simulink model "PI_PSO"  (R2021a)
settings: Solver=VariableStepAuto  StartTime=0.0  StopTime=100  RelTol=1e-6  AbsTol=1e-6
undefined symbols (not defined in the file or in its folder): DiscIntNeverNeededParam, G, Solar_time, wind, wind_time
libraries: powerlib_extras x24, pid_lib x6, simulink x2
(part 2 of 2)

== system PI_PSO/AREA 2/Performance Indices/ITSE ==
  In1 : Inport
  Clock : Clock
  Discrete-Time Integrator : DiscreteIntegrator  gainval=1  SampleTime=-1  ICPrevOutput=DiscIntNeverNeededParam  ICPrevScaledInput=DiscIntNeverNeededParam
  Divide : Product  Inputs=**
  Math Function : Math  Operator=square  SignedPower=on  SaturateOnIntegerOverflow=on
  Out1 : Outport
  wires:
  Discrete-Time Integrator/1 -> Out1/1
  In1/1 -> Math Function/1
  Divide/1 -> Discrete-Time Integrator/1
  Math Function/1 -> Divide/1
  Clock/1 -> Divide/2

== system PI_PSO/AREA 2/Performance Indices/Subsystem1 ==
  In1 : Inport
  Id_ref step : powerlib_extras/Control  Blocks/Timer  t=[0 1]  e=[0 1]
      settings: SourceProductBaseCode=PS
  Prod : Product  InputSameDT=on  SaturateOnIntegerOverflow=on  OutDataTypeStr=Inherit: Same as first input
  DP1 : Outport
  wires:
  Id_ref step/1 -> Prod/2
  In1/1 -> Prod/1
  Prod/1 -> DP1/1

== system PI_PSO/AREA 2/Performance Indices/Subsystem2 ==
  In1 : Inport
  Id_ref step : powerlib_extras/Control  Blocks/Timer  t=[0 1]  e=[0 1]
      settings: SourceProductBaseCode=PS
  Prod : Product  InputSameDT=on  SaturateOnIntegerOverflow=on  OutDataTypeStr=Inherit: Same as first input
  Out1 : Outport
  wires:
  Id_ref step/1 -> Prod/2
  In1/1 -> Prod/1
  Prod/1 -> Out1/1

== system PI_PSO/AREA 2/Performance Indices/Subsystem3 ==
  In1 : Inport
  Id_ref step : powerlib_extras/Control  Blocks/Timer  t=[0 1]  e=[0 1]
      settings: SourceProductBaseCode=PS
  Prod : Product  InputSameDT=on  SaturateOnIntegerOverflow=on  OutDataTypeStr=Inherit: Same as first input
  Out1 : Outport
  wires:
  Prod/1 -> Out1/1
  In1/1 -> Prod/1
  Id_ref step/1 -> Prod/2

== system PI_PSO/AREA 2/Performance Indices/Subsystem5 ==
  In1 : Inport
  Id_ref step : powerlib_extras/Control  Blocks/Timer  t=[0 1]  e=[0 1]
      settings: SourceProductBaseCode=PS
  Prod : Product  InputSameDT=on  SaturateOnIntegerOverflow=on  OutDataTypeStr=Inherit: Same as first input
  Out1 : Outport
  wires:
  Prod/1 -> Out1/1
  In1/1 -> Prod/1
  Id_ref step/1 -> Prod/2

== system PI_PSO/AREA 3/Performance Indices/IAE ==
  In1 : Inport
  Abs : Abs
  Discrete-Time Integrator : DiscreteIntegrator  gainval=1  SampleTime=-1  ICPrevOutput=DiscIntNeverNeededParam  ICPrevScaledInput=DiscIntNeverNeededParam
  Out1 : Outport
  wires:
  Abs/1 -> Discrete-Time Integrator/1
  Discrete-Time Integrator/1 -> Out1/1
  In1/1 -> Abs/1

== system PI_PSO/AREA 3/Performance Indices/ISE ==
  In1 : Inport
  Discrete-Time Integrator : DiscreteIntegrator  gainval=1  SampleTime=-1  ICPrevOutput=DiscIntNeverNeededParam  ICPrevScaledInput=DiscIntNeverNeededParam
  Math Function : Math  Operator=square  SignedPower=on  SaturateOnIntegerOverflow=on
  Out1 : Outport
  wires:
  In1/1 -> Math Function/1
  Discrete-Time Integrator/1 -> Out1/1
  Math Function/1 -> Discrete-Time Integrator/1

== system PI_PSO/AREA 3/Performance Indices/ITAE2 ==
  In1 : Inport
  Abs : Abs
  Clock : Clock
  Discrete-Time Integrator : DiscreteIntegrator  gainval=1  SampleTime=-1  ICPrevOutput=DiscIntNeverNeededParam  ICPrevScaledInput=DiscIntNeverNeededParam
  Divide : Product  Inputs=**
  Out1 : Outport
  wires:
  Clock/1 -> Divide/2
  Abs/1 -> Divide/1
  Divide/1 -> Discrete-Time Integrator/1
  In1/1 -> Abs/1
  Discrete-Time Integrator/1 -> Out1/1

== system PI_PSO/AREA 3/Performance Indices/ITSE ==
  In1 : Inport
  Clock : Clock
  Discrete-Time Integrator : DiscreteIntegrator  gainval=1  SampleTime=-1  ICPrevOutput=DiscIntNeverNeededParam  ICPrevScaledInput=DiscIntNeverNeededParam
  Divide : Product  Inputs=**
  Math Function : Math  Operator=square  SignedPower=on  SaturateOnIntegerOverflow=on
  Out1 : Outport
  wires:
  Discrete-Time Integrator/1 -> Out1/1
  In1/1 -> Math Function/1
  Divide/1 -> Discrete-Time Integrator/1
  Math Function/1 -> Divide/1
  Clock/1 -> Divide/2

== system PI_PSO/AREA 3/Performance Indices/Subsystem1 ==
  In1 : Inport
  Id_ref step : powerlib_extras/Control  Blocks/Timer  t=[0 1]  e=[0 1]
      settings: SourceProductBaseCode=PS
  Prod : Product  InputSameDT=on  SaturateOnIntegerOverflow=on  OutDataTypeStr=Inherit: Same as first input
  Out1 : Outport
  wires:
  Id_ref step/1 -> Prod/2
  In1/1 -> Prod/1
  Prod/1 -> Out1/1

== system PI_PSO/AREA 3/Performance Indices/Subsystem2 ==
  In1 : Inport
  Id_ref step : powerlib_extras/Control  Blocks/Timer  t=[0 1]  e=[0 1]
      settings: SourceProductBaseCode=PS
  Prod : Product  InputSameDT=on  SaturateOnIntegerOverflow=on  OutDataTypeStr=Inherit: Same as first input
  DP1 : Outport
  wires:
  Id_ref step/1 -> Prod/2
  In1/1 -> Prod/1
  Prod/1 -> DP1/1

== system PI_PSO/AREA 3/Performance Indices/Subsystem3 ==
  In1 : Inport
  Id_ref step : powerlib_extras/Control  Blocks/Timer  t=[0 1]  e=[0 1]
      settings: SourceProductBaseCode=PS
  Prod : Product  InputSameDT=on  SaturateOnIntegerOverflow=on  OutDataTypeStr=Inherit: Same as first input
  Out1 : Outport
  wires:
  Prod/1 -> Out1/1
  In1/1 -> Prod/1
  Id_ref step/1 -> Prod/2

== system PI_PSO/AREA 3/Performance Indices/Subsystem5 ==
  In1 : Inport
  Id_ref step : powerlib_extras/Control  Blocks/Timer  t=[0 1]  e=[0 1]
      settings: SourceProductBaseCode=PS
  Prod : Product  InputSameDT=on  SaturateOnIntegerOverflow=on  OutDataTypeStr=Inherit: Same as first input
  Out1 : Outport
  wires:
  Prod/1 -> Out1/1
  In1/1 -> Prod/1
  Id_ref step/1 -> Prod/2

== system PI_PSO/AREA 4/Performance Indices/IAE ==
  In1 : Inport
  Abs : Abs
  Discrete-Time Integrator : DiscreteIntegrator  gainval=1  SampleTime=-1  ICPrevOutput=DiscIntNeverNeededParam  ICPrevScaledInput=DiscIntNeverNeededParam
  Out1 : Outport
  wires:
  Abs/1 -> Discrete-Time Integrator/1
  Discrete-Time Integrator/1 -> Out1/1
  In1/1 -> Abs/1

== system PI_PSO/AREA 4/Performance Indices/ISE ==
  In1 : Inport
  Discrete-Time Integrator : DiscreteIntegrator  gainval=1  SampleTime=-1  ICPrevOutput=DiscIntNeverNeededParam  ICPrevScaledInput=DiscIntNeverNeededParam
  Math Function : Math  Operator=square  SignedPower=on  SaturateOnIntegerOverflow=on
  Out1 : Outport
  wires:
  In1/1 -> Math Function/1
  Discrete-Time Integrator/1 -> Out1/1
  Math Function/1 -> Discrete-Time Integrator/1

== system PI_PSO/AREA 4/Performance Indices/ITAE4 ==
  In1 : Inport
  Abs : Abs
  Clock : Clock
  Discrete-Time Integrator : DiscreteIntegrator  gainval=1  SampleTime=-1  ICPrevOutput=DiscIntNeverNeededParam  ICPrevScaledInput=DiscIntNeverNeededParam
  Divide : Product  Inputs=**
  Out1 : Outport
  wires:
  Clock/1 -> Divide/2
  Abs/1 -> Divide/1
  Divide/1 -> Discrete-Time Integrator/1
  In1/1 -> Abs/1
  Discrete-Time Integrator/1 -> Out1/1

== system PI_PSO/AREA 4/Performance Indices/ITSE ==
  In1 : Inport
  Clock : Clock
  Discrete-Time Integrator : DiscreteIntegrator  gainval=1  SampleTime=-1  ICPrevOutput=DiscIntNeverNeededParam  ICPrevScaledInput=DiscIntNeverNeededParam
  Divide : Product  Inputs=**
  Math Function : Math  Operator=square  SignedPower=on  SaturateOnIntegerOverflow=on
  Out1 : Outport
  wires:
  Discrete-Time Integrator/1 -> Out1/1
  In1/1 -> Math Function/1
  Divide/1 -> Discrete-Time Integrator/1
  Math Function/1 -> Divide/1
  Clock/1 -> Divide/2

== system PI_PSO/AREA 4/Performance Indices/Subsystem1 ==
  In1 : Inport
  Id_ref step : powerlib_extras/Control  Blocks/Timer  t=[0 1]  e=[0 1]
      settings: SourceProductBaseCode=PS
  Prod : Product  InputSameDT=on  SaturateOnIntegerOverflow=on  OutDataTypeStr=Inherit: Same as first input
  Out1 : Outport
  wires:
  Id_ref step/1 -> Prod/2
  In1/1 -> Prod/1
  Prod/1 -> Out1/1

== system PI_PSO/AREA 4/Performance Indices/Subsystem2 ==
  In1 : Inport
  Id_ref step : powerlib_extras/Control  Blocks/Timer  t=[0 1]  e=[0 1]
      settings: SourceProductBaseCode=PS
  Prod : Product  InputSameDT=on  SaturateOnIntegerOverflow=on  OutDataTypeStr=Inherit: Same as first input
  Out1 : Outport
  wires:
  Prod/1 -> Out1/1
  In1/1 -> Prod/1
  Id_ref step/1 -> Prod/2

== system PI_PSO/AREA 4/Performance Indices/Subsystem3 ==
  In1 : Inport
  Id_ref step : powerlib_extras/Control  Blocks/Timer  t=[0 1]  e=[0 1]
      settings: SourceProductBaseCode=PS
  Prod : Product  InputSameDT=on  SaturateOnIntegerOverflow=on  OutDataTypeStr=Inherit: Same as first input
  DP1 : Outport
  wires:
  Id_ref step/1 -> Prod/2
  In1/1 -> Prod/1
  Prod/1 -> DP1/1

== system PI_PSO/AREA 4/Performance Indices/Subsystem5 ==
  In1 : Inport
  Id_ref step : powerlib_extras/Control  Blocks/Timer  t=[0 1]  e=[0 1]
      settings: SourceProductBaseCode=PS
  Prod : Product  InputSameDT=on  SaturateOnIntegerOverflow=on  OutDataTypeStr=Inherit: Same as first input
  Out1 : Outport
  wires:
  Prod/1 -> Out1/1
  In1/1 -> Prod/1
  Id_ref step/1 -> Prod/2

== system PI_PSO/AREA 5/Performance Indices/IAE ==
  In1 : Inport
  Abs : Abs
  Discrete-Time Integrator : DiscreteIntegrator  gainval=1  SampleTime=-1  ICPrevOutput=DiscIntNeverNeededParam  ICPrevScaledInput=DiscIntNeverNeededParam
  Out1 : Outport
  wires:
  Abs/1 -> Discrete-Time Integrator/1
  Discrete-Time Integrator/1 -> Out1/1
  In1/1 -> Abs/1

== system PI_PSO/AREA 5/Performance Indices/ISE ==
  In1 : Inport
  Discrete-Time Integrator : DiscreteIntegrator  gainval=1  SampleTime=-1  ICPrevOutput=DiscIntNeverNeededParam  ICPrevScaledInput=DiscIntNeverNeededParam
  Math Function : Math  Operator=square  SignedPower=on  SaturateOnIntegerOverflow=on
  Out1 : Outport
  wires:
  In1/1 -> Math Function/1
  Discrete-Time Integrator/1 -> Out1/1
  Math Function/1 -> Discrete-Time Integrator/1

== system PI_PSO/AREA 5/Performance Indices/ITAE5 ==
  In1 : Inport
  Abs : Abs
  Clock : Clock
  Discrete-Time Integrator : DiscreteIntegrator  gainval=1  SampleTime=-1  ICPrevOutput=DiscIntNeverNeededParam  ICPrevScaledInput=DiscIntNeverNeededParam
  Divide : Product  Inputs=**
  Out1 : Outport
  wires:
  Clock/1 -> Divide/2
  Abs/1 -> Divide/1
  Divide/1 -> Discrete-Time Integrator/1
  In1/1 -> Abs/1
  Discrete-Time Integrator/1 -> Out1/1

== system PI_PSO/AREA 5/Performance Indices/ITSE ==
  In1 : Inport
  Clock : Clock
  Discrete-Time Integrator : DiscreteIntegrator  gainval=1  SampleTime=-1  ICPrevOutput=DiscIntNeverNeededParam  ICPrevScaledInput=DiscIntNeverNeededParam
  Divide : Product  Inputs=**
  Math Function : Math  Operator=square  SignedPower=on  SaturateOnIntegerOverflow=on
  Out1 : Outport
  wires:
  Discrete-Time Integrator/1 -> Out1/1
  In1/1 -> Math Function/1
  Divide/1 -> Discrete-Time Integrator/1
  Math Function/1 -> Divide/1
  Clock/1 -> Divide/2

== system PI_PSO/AREA 5/Performance Indices/Subsystem1 ==
  In1 : Inport
  Id_ref step : powerlib_extras/Control  Blocks/Timer  t=[0 1]  e=[0 1]
      settings: SourceProductBaseCode=PS
  Prod : Product  InputSameDT=on  SaturateOnIntegerOverflow=on  OutDataTypeStr=Inherit: Same as first input
  Out1 : Outport
  wires:
  Id_ref step/1 -> Prod/2
  In1/1 -> Prod/1
  Prod/1 -> Out1/1

== system PI_PSO/AREA 5/Performance Indices/Subsystem2 ==
  In1 : Inport
  Id_ref step : powerlib_extras/Control  Blocks/Timer  t=[0 1]  e=[0 1]
      settings: SourceProductBaseCode=PS
  Prod : Product  InputSameDT=on  SaturateOnIntegerOverflow=on  OutDataTypeStr=Inherit: Same as first input
  Out1 : Outport
  wires:
  Prod/1 -> Out1/1
  In1/1 -> Prod/1
  Id_ref step/1 -> Prod/2

== system PI_PSO/AREA 5/Performance Indices/Subsystem3 ==
  In1 : Inport
  Id_ref step : powerlib_extras/Control  Blocks/Timer  t=[0 1]  e=[0 1]
      settings: SourceProductBaseCode=PS
  Prod : Product  InputSameDT=on  SaturateOnIntegerOverflow=on  OutDataTypeStr=Inherit: Same as first input
  Out1 : Outport
  wires:
  Prod/1 -> Out1/1
  In1/1 -> Prod/1
  Id_ref step/1 -> Prod/2

== system PI_PSO/AREA 5/Performance Indices/Subsystem5 ==
  In1 : Inport
  Id_ref step : powerlib_extras/Control  Blocks/Timer  t=[0 1]  e=[0 1]
      settings: SourceProductBaseCode=PS
  Prod : Product  InputSameDT=on  SaturateOnIntegerOverflow=on  OutDataTypeStr=Inherit: Same as first input
  DP1 : Outport
  wires:
  Id_ref step/1 -> Prod/2
  In1/1 -> Prod/1
  Prod/1 -> DP1/1

== system PI_PSO/AREA 6/Performance Indices/IAE ==
  In1 : Inport
  Abs : Abs
  Discrete-Time Integrator : DiscreteIntegrator  gainval=1  SampleTime=-1  ICPrevOutput=DiscIntNeverNeededParam  ICPrevScaledInput=DiscIntNeverNeededParam
  Out1 : Outport
  wires:
  Abs/1 -> Discrete-Time Integrator/1
  Discrete-Time Integrator/1 -> Out1/1
  In1/1 -> Abs/1

== system PI_PSO/AREA 6/Performance Indices/ISE ==
  In1 : Inport
  Discrete-Time Integrator : DiscreteIntegrator  gainval=1  SampleTime=-1  ICPrevOutput=DiscIntNeverNeededParam  ICPrevScaledInput=DiscIntNeverNeededParam
  Math Function : Math  Operator=square  SignedPower=on  SaturateOnIntegerOverflow=on
  Out1 : Outport
  wires:
  In1/1 -> Math Function/1
  Discrete-Time Integrator/1 -> Out1/1
  Math Function/1 -> Discrete-Time Integrator/1

== system PI_PSO/AREA 6/Performance Indices/ITAE6 ==
  In1 : Inport
  Abs : Abs
  Clock : Clock
  Discrete-Time Integrator : DiscreteIntegrator  gainval=1  SampleTime=-1  ICPrevOutput=DiscIntNeverNeededParam  ICPrevScaledInput=DiscIntNeverNeededParam
  Divide : Product  Inputs=**
  Out1 : Outport
  wires:
  Clock/1 -> Divide/2
  Abs/1 -> Divide/1
  Divide/1 -> Discrete-Time Integrator/1
  In1/1 -> Abs/1
  Discrete-Time Integrator/1 -> Out1/1

== system PI_PSO/AREA 6/Performance Indices/ITSE ==
  In1 : Inport
  Clock : Clock
  Discrete-Time Integrator : DiscreteIntegrator  gainval=1  SampleTime=-1  ICPrevOutput=DiscIntNeverNeededParam  ICPrevScaledInput=DiscIntNeverNeededParam
  Divide : Product  Inputs=**
  Math Function : Math  Operator=square  SignedPower=on  SaturateOnIntegerOverflow=on
  Out1 : Outport
  wires:
  Discrete-Time Integrator/1 -> Out1/1
  In1/1 -> Math Function/1
  Divide/1 -> Discrete-Time Integrator/1
  Math Function/1 -> Divide/1
  Clock/1 -> Divide/2

== system PI_PSO/AREA 6/Performance Indices/Subsystem1 ==
  In1 : Inport
  Id_ref step : powerlib_extras/Control  Blocks/Timer  t=[0 1]  e=[0 1]
      settings: SourceProductBaseCode=PS
  Prod : Product  InputSameDT=on  SaturateOnIntegerOverflow=on  OutDataTypeStr=Inherit: Same as first input
  Out1 : Outport
  wires:
  Id_ref step/1 -> Prod/2
  In1/1 -> Prod/1
  Prod/1 -> Out1/1

== system PI_PSO/AREA 6/Performance Indices/Subsystem2 ==
  In1 : Inport
  Id_ref step : powerlib_extras/Control  Blocks/Timer  t=[0 1]  e=[0 1]
      settings: SourceProductBaseCode=PS
  Prod : Product  InputSameDT=on  SaturateOnIntegerOverflow=on  OutDataTypeStr=Inherit: Same as first input
  Out1 : Outport
  wires:
  Prod/1 -> Out1/1
  In1/1 -> Prod/1
  Id_ref step/1 -> Prod/2

== system PI_PSO/AREA 6/Performance Indices/Subsystem5 ==
  In1 : Inport
  Id_ref step : powerlib_extras/Control  Blocks/Timer  t=[0 1]  e=[0 1]
      settings: SourceProductBaseCode=PS
  Prod : Product  InputSameDT=on  SaturateOnIntegerOverflow=on  OutDataTypeStr=Inherit: Same as first input
  Out1 : Outport
  wires:
  Prod/1 -> Out1/1
  In1/1 -> Prod/1
  Id_ref step/1 -> Prod/2

== system PI_PSO/AREA 6/Performance Indices/Subsystem6 ==
  In1 : Inport
  Id_ref step : powerlib_extras/Control  Blocks/Timer  t=[0 1]  e=[0 1]
      settings: SourceProductBaseCode=PS
  Prod : Product  InputSameDT=on  SaturateOnIntegerOverflow=on  OutDataTypeStr=Inherit: Same as first input
  DP1 : Outport
  wires:
  Id_ref step/1 -> Prod/2
  In1/1 -> Prod/1
  Prod/1 -> DP1/1

== system PI_PSO/SWITCH CASE/SWITCH CASE/Load decrement Only ==
  Action Port : ActionPort  ActionPortLabel=case [ 4 ]:
  Clock : Clock
  Compare To Constant : simulink/Logic and Bit Operations/Compare To Constant  relop=>=  const=15  OutDataTypeStr=boolean
  Subsystem : Subsystem
  " " : Outport
  "L2 " : Outport  Port=2
  "L3 " : Outport  Port=3
  "L4 " : Outport  Port=4
  "L5 " : Outport  Port=5
  "L6 " : Outport  Port=6
  wires:
  Subsystem/3(Out3) -> "L3 "/1
  Clock/1 -> Compare To Constant/1
  Subsystem/1(Out1) -> " "/1
  Subsystem/6(Out6) -> "L6 "/1
  Subsystem/4(Out4) -> "L4 "/1
  Subsystem/2(Out2) -> "L2 "/1
  Compare To Constant/1 -> Subsystem/Trigger
  Subsystem/5(Out5) -> "L5 "/1

== system PI_PSO/SWITCH CASE/SWITCH CASE/PV + WIND  ==
  Action Port : ActionPort  ActionPortLabel=case [ 2 ]:
  "PV Farm " : Subsystem
      mask Display: image('panel.jpg')
  "Wind Farm " : Subsystem
      mask Display: image('windfarm.jpg')
  "PV_Farm " : Outport
  "Wind_Farm " : Outport  Port=2
  wires:
  "PV Farm "/1(P_Solar) -> "PV_Farm "/1
  "Wind Farm "/1(P_wind) -> "Wind_Farm "/1

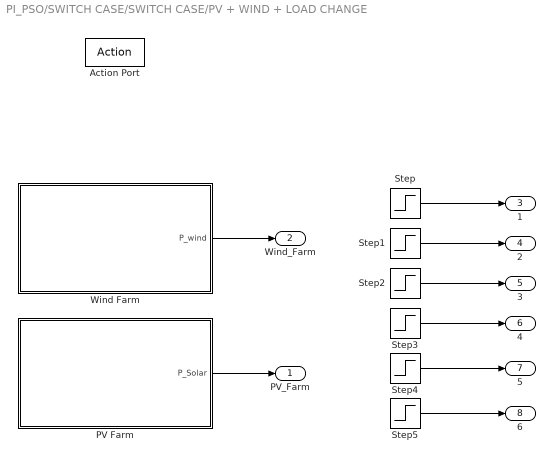
== system PI_PSO/SWITCH CASE/SWITCH CASE/PV + WIND + LOAD CHANGE ==
  Action Port : ActionPort  ActionPortLabel=case [ 5 ]:
  "PV Farm " : Subsystem
      mask Display: image('panel.jpg')
  Step{,1..5} (6 alike) : Step  Time=100  Before=0.1  After=0.1  SampleTime=0
  "Wind Farm " : Subsystem
      mask Display: image('windfarm.jpg')
  "PV_Farm " : Outport
  "Wind_Farm " : Outport  Port=2
  "1 " : Outport  Port=3
  "2 " : Outport  Port=4
  "3 " : Outport  Port=5
  4 : Outport  Port=6
  "5 " : Outport  Port=7
  "6 " : Outport  Port=8
  wires:
  Step/1 -> "1 "/1
  "PV Farm "/1(P_Solar) -> "PV_Farm "/1
  "Wind Farm "/1(P_wind) -> "Wind_Farm "/1
  Step1/1 -> "2 "/1
  Step2/1 -> "3 "/1
  Step3/1 -> 4/1
  Step4/1 -> "5 "/1
  Step5/1 -> "6 "/1

== system PI_PSO/SWITCH CASE/SWITCH CASE/PV Only ==
  Action Port : ActionPort  ActionPortLabel=case [ 1 ]:
  "PV Farm " : Subsystem
      mask Display: image('panel.jpg')
  "PV ONLY " : Outport
  wires:
  "PV Farm "/1(P_Solar) -> "PV ONLY "/1

== system PI_PSO/SWITCH CASE/SWITCH CASE/Switch Case Action Subsystem5 ==
  Action Port : ActionPort  ActionPortLabel=case [ 3 ]:
  Clock : Clock
  Compare To Constant : simulink/Logic and Bit Operations/Compare To Constant  relop=>=  const=15  OutDataTypeStr=boolean
  Subsystem : Subsystem
  "L2 " : Outport
  "L4 " : Outport  Port=2
  "L6 " : Outport  Port=3
  wires:
  Subsystem/2("4 ") -> "L4 "/1
  Subsystem/1(2) -> "L2 "/1
  Clock/1 -> Compare To Constant/1
  Compare To Constant/1 -> Subsystem/Trigger
  Subsystem/3("6 ") -> "L6 "/1

== system PI_PSO/SWITCH CASE/SWITCH CASE/WIND Only ==
  Action Port : ActionPort  ActionPortLabel=case [ 0 ]:
  "Wind Farm " : Subsystem
      mask Display: image('windfarm.jpg')
  "Wind Farm ONLY " : Outport
  wires:
  "Wind Farm "/1(P_wind) -> "Wind Farm ONLY "/1

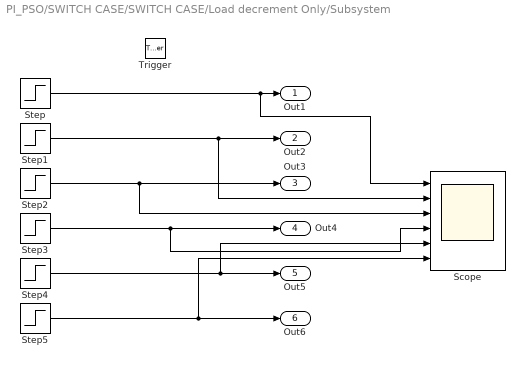
== system PI_PSO/SWITCH CASE/SWITCH CASE/Load decrement Only/Subsystem ==
  Trigger : TriggerPort  VariantControl=(inherit)  PortDimensions=1
  Scope : Scope  NumInputPorts=6
  Step{,1..5} (6 alike) : Step  Time=100  Before=0.1  After=0.1
  Out1 : Outport
  Out2 : Outport  Port=2
  Out3 : Outport  Port=3
  Out4 : Outport  Port=4
  Out5 : Outport  Port=5
  Out6 : Outport  Port=6
  wires:
  Step3/1 -> Scope/4, Out4/1
  Step5/1 -> Scope/6, Out6/1
  Step1/1 -> Scope/2, Out2/1
  Step2/1 -> Scope/3, Out3/1
  Step/1 -> Scope/1, Out1/1
  Step4/1 -> Scope/5, Out5/1

== system PI_PSO/SWITCH CASE/SWITCH CASE/PV + WIND /PV Farm  ==
  Irradiance : Subsystem
      mask init:
      | load power_V2G
      mask Display: plot(V2G.IRRADIANCE.time,V2G.IRRADIANCE.SUN)
  Solar Farm : TransferFcn  Numerator=[0.8]  Denominator=[0.8 1]
  P_Solar : Outport
  wires:
  Solar Farm/1 -> P_Solar/1
  Irradiance/1(" ") -> Solar Farm/1

== system PI_PSO/SWITCH CASE/SWITCH CASE/PV + WIND /Wind Farm  ==
  WInd Farm : TransferFcn  Denominator=[0.9 1]
  Wind profile : Subsystem
      mask init:
      | load power_V2G
      mask Display: plot(V2G.WINDTURBINE.time,V2G.WINDTURBINE.wind)
  P_wind : Outport
  wires:
  Wind profile/1(" ") -> WInd Farm/1
  WInd Farm/1 -> P_wind/1

== system PI_PSO/SWITCH CASE/SWITCH CASE/PV + WIND + LOAD CHANGE/PV Farm  ==
  Irradiance : Subsystem
      mask init:
      | load power_V2G
      mask Display: plot(V2G.IRRADIANCE.time,V2G.IRRADIANCE.SUN)
  Solar Farm : TransferFcn  Numerator=[0.8]  Denominator=[0.8 1]
  P_Solar : Outport
  wires:
  Irradiance/1(" ") -> Solar Farm/1
  Solar Farm/1 -> P_Solar/1

== system PI_PSO/SWITCH CASE/SWITCH CASE/PV + WIND + LOAD CHANGE/Wind Farm  ==
  WInd Farm : TransferFcn  Denominator=[0.9 1]
  Wind profile : Subsystem
      mask init:
      | load power_V2G
      mask Display: plot(V2G.WINDTURBINE.time,V2G.WINDTURBINE.wind)
  P_wind : Outport
  wires:
  WInd Farm/1 -> P_wind/1
  Wind profile/1(" ") -> WInd Farm/1

== system PI_PSO/SWITCH CASE/SWITCH CASE/PV Only/PV Farm  ==
  Irradiance : Subsystem
      mask init:
      | load power_V2G
      mask Display: plot(V2G.IRRADIANCE.time,V2G.IRRADIANCE.SUN)
  Solar Farm : TransferFcn  Numerator=[0.8]  Denominator=[0.8 1]
  P_Solar : Outport
  wires:
  Irradiance/1(" ") -> Solar Farm/1
  Solar Farm/1 -> P_Solar/1

== system PI_PSO/SWITCH CASE/SWITCH CASE/Switch Case Action Subsystem5/Subsystem ==
  Trigger : TriggerPort  VariantControl=(inherit)  PortDimensions=1
  Scope : Scope  NumInputPorts=6
  Step1 : Step  Time=100  Before=0.1  After=0.1
  Step3 : Step  Time=100  Before=0.2  After=0.2
  Step5 : Step  Time=100  Before=0.3  After=0.3
  2 : Outport
  "4 " : Outport  Port=2
  "6 " : Outport  Port=3
  wires:
  Step3/1 -> Scope/4, "4 "/1
  Step5/1 -> Scope/6, "6 "/1
  Step1/1 -> Scope/2, 2/1

== system PI_PSO/SWITCH CASE/SWITCH CASE/WIND Only/Wind Farm  ==
  WInd Farm : TransferFcn  Denominator=[0.9 1]
  Wind profile : Subsystem
      mask init:
      | load power_V2G
      mask Display: plot(V2G.WINDTURBINE.time,V2G.WINDTURBINE.wind)
  P_wind : Outport
  wires:
  Wind profile/1(" ") -> WInd Farm/1
  WInd Farm/1 -> P_wind/1

== system PI_PSO/SWITCH CASE/SWITCH CASE/PV + WIND /PV Farm /Irradiance ==
  1-D Lookup Table : Lookup_n-D  NumberOfTableDimensions=1  BreakpointsForDimension1=Solar_time  Table=G  InternalRulePriority=Speed  RndMeth=Simplest  InputSameDT=on
  Clock1 : Clock
  " " : Outport  VectorParamsAs1DForOutWhenUnconnected=off
  wires:
  Clock1/1 -> 1-D Lookup Table/1
  1-D Lookup Table/1 -> " "/1

== system PI_PSO/SWITCH CASE/SWITCH CASE/PV + WIND /Wind Farm /Wind profile ==
  1-D Lookup Table1 : Lookup_n-D  NumberOfTableDimensions=1  BreakpointsForDimension1=wind_time  Table=wind  InternalRulePriority=Speed  RndMeth=Simplest  InputSameDT=on
  Clock1 : Clock
  " " : Outport  VectorParamsAs1DForOutWhenUnconnected=off
  wires:
  Clock1/1 -> 1-D Lookup Table1/1
  1-D Lookup Table1/1 -> " "/1

== system PI_PSO/SWITCH CASE/SWITCH CASE/PV + WIND + LOAD CHANGE/PV Farm /Irradiance ==
  1-D Lookup Table : Lookup_n-D  NumberOfTableDimensions=1  BreakpointsForDimension1=Solar_time  Table=G  InternalRulePriority=Speed  RndMeth=Simplest  InputSameDT=on
  Clock1 : Clock
  " " : Outport  VectorParamsAs1DForOutWhenUnconnected=off
  wires:
  1-D Lookup Table/1 -> " "/1
  Clock1/1 -> 1-D Lookup Table/1

== system PI_PSO/SWITCH CASE/SWITCH CASE/PV + WIND + LOAD CHANGE/Wind Farm /Wind profile ==
  1-D Lookup Table1 : Lookup_n-D  NumberOfTableDimensions=1  BreakpointsForDimension1=wind_time  Table=wind  InternalRulePriority=Speed  RndMeth=Simplest  InputSameDT=on
  Clock1 : Clock
  " " : Outport  VectorParamsAs1DForOutWhenUnconnected=off
  wires:
  1-D Lookup Table1/1 -> " "/1
  Clock1/1 -> 1-D Lookup Table1/1

== system PI_PSO/SWITCH CASE/SWITCH CASE/PV Only/PV Farm /Irradiance ==
  1-D Lookup Table : Lookup_n-D  NumberOfTableDimensions=1  BreakpointsForDimension1=Solar_time  Table=G  InternalRulePriority=Speed  RndMeth=Simplest  InputSameDT=on
  Clock1 : Clock
  " " : Outport  VectorParamsAs1DForOutWhenUnconnected=off
  wires:
  1-D Lookup Table/1 -> " "/1
  Clock1/1 -> 1-D Lookup Table/1

== system PI_PSO/SWITCH CASE/SWITCH CASE/WIND Only/Wind Farm /Wind profile ==
  1-D Lookup Table1 : Lookup_n-D  NumberOfTableDimensions=1  BreakpointsForDimension1=wind_time  Table=wind  InternalRulePriority=Speed  RndMeth=Simplest  InputSameDT=on
  Clock1 : Clock
  " " : Outport  VectorParamsAs1DForOutWhenUnconnected=off
  wires:
  Clock1/1 -> 1-D Lookup Table1/1
  1-D Lookup Table1/1 -> " "/1
